simulink model "Mag_VarAeroBlock"  (R2016b)
settings: Solver=VariableStepAuto  StartTime=0.0  StopTime=10.0  RelTol=1e-3
undefined symbols (not defined in the file or in its folder): Env, Sim
libraries: aerolibobsolete x1
settings Model: Creator=rega0051  LastModifiedBy=rega0051
settings DataIOCC: SaveOutput=off  SignalLogging=off  DSMLogging=off  SaveTime=off

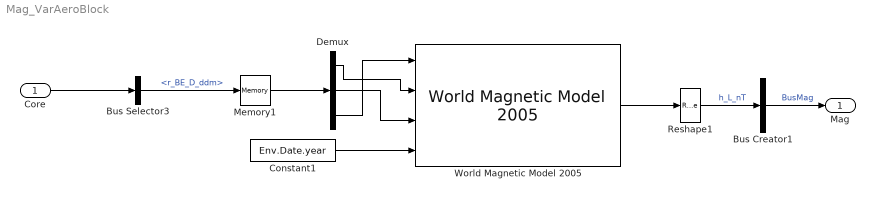
== system Mag_VarAeroBlock ==
  Core : Inport  OutDataTypeStr=Bus: BusCore
      settings: AttributesFormatString=%<OutDataTypeStr>
  Bus Creator1 : BusCreator  Inputs=1  OutDataTypeStr=Bus: BusMag
      settings: AttributesFormatString=%<OutDataTypeStr>  InheritFromInputs=off
  Bus Selector3 : BusSelector  OutputSignals=BusEom.r_BE_D_ddm
  Constant1 : Constant  Value=Env.Date.year
      settings: AttributesFormatString=%<Value>
  Demux : Demux  Outputs=3
  Memory1 : Memory  X0=Sim.Trim.Init.rInit_BE_D_ddm  InheritSampleTime=on  LinearizeMemory=on  LinearizeAsDelay=on
      settings: AttributesFormatString=%<X0>
  Reshape1 : Reshape  OutputDimensionality=Column vector (2-D)  OutputDimensions=[3,1]
  World Magnetic Model 2005 : aerolibobsolete/World Magnetic Model 2005  units=Metric (MKS)  time_in=on  month=January  day=1  year=2005  action=None  h_out=off  dec_out=off  inc_out=off  ti_out=off
  Mag : Outport  OutDataTypeStr=Bus: BusMag
      settings: AttributesFormatString=%<OutDataTypeStr>
  wires:
  Memory1/1 -> Demux/1
  Bus Selector3/1 -> Memory1/1  "<r_BE_D_ddm>"
  Reshape1/1 -> Bus Creator1/1  "h_L_nT"
  Core/1 -> Bus Selector3/1
  Demux/1 -> World Magnetic Model 2005/2
  Demux/2 -> World Magnetic Model 2005/3
  Demux/3 -> World Magnetic Model 2005/1
  Constant1/1 -> World Magnetic Model 2005/4
  World Magnetic Model 2005/1 -> Reshape1/1
  Bus Creator1/1 -> Mag/1  "BusMag"
